simulink model "diagram"  (R2024b)
settings: Solver=VariableStepAuto  StartTime=0.0  StopTime=10.0  RelTol=1e-3
libraries: simulink x1
settings Model: Creator=Okuyt  LastModifiedBy=Okuyt

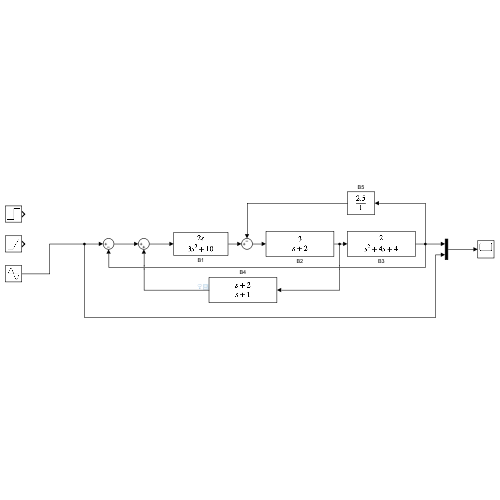
[thumbnail: Simulink's stored preview of the top-level diagram]
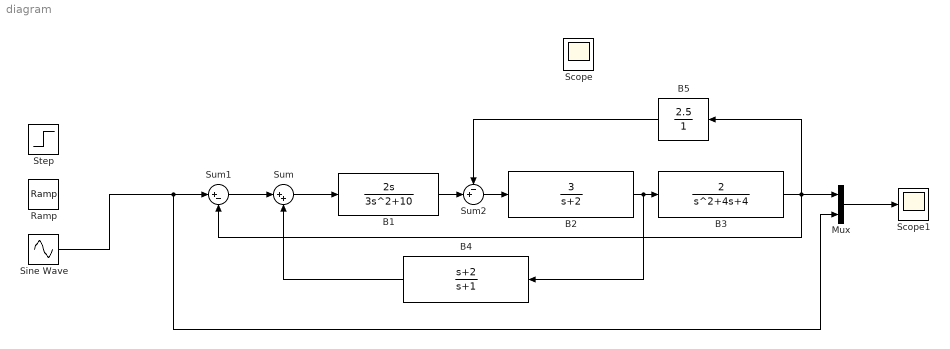
== system diagram ==
  B1 : TransferFcn  Numerator=[2 0]  Denominator=[3 0 10]
  B2 : TransferFcn  Numerator=[3]  Denominator=[1 2]
  B3 : TransferFcn  Numerator=[2]  Denominator=[1 4 4]
  B4 : TransferFcn  Numerator=[1 2]  Denominator=[1 1]
  B5 : TransferFcn  Numerator=[2.5]  Denominator=[1]
  Mux : Mux  Inputs=2
  Ramp : simulink/Sources/Ramp  slope=1  start=0  InitialOutput=0
  Scope1 : Scope
  Sine Wave : Sin  SampleTime=0
  Step : Step  SampleTime=0
  Sum : Sum  Inputs=|++
  Sum1 : Sum  Inputs=|+-
  Sum2 : Sum  Inputs=-+|
  Scope : Scope
  wires:
  Sum1/1 -> Sum/1
  B1/1 -> Sum2/2
  Sum2/1 -> B2/1
  B2/1 -> B4/1, B3/1
  B3/1 -> B5/1, Mux/1, Sum1/2
  B4/1 -> Sum/2
  Sine Wave/1 -> Mux/2, Sum1/1
  Sum/1 -> B1/1
  Mux/1 -> Scope1/1
  B5/1 -> Sum2/1
